simulink model "IEEE34bus_v2019b_Phasor_DPL_ZIPload"  (R2019b)
settings: Solver=VariableStepAuto  StartTime=0.0  StopTime=100  FixedStep=Ts  RelTol=1e-3
InitFcn:
  | a=1; % Loading Factor
  | Ts=0.1;% For Delay Blocks in Voltage Regulator Controls
  | 
  | % Simulation data for the IEEE 34 Node Test Feeder model
  | mi2km = 1.60934;%  miles to km conversion
  | ft2km = 0.0003048; % feet to km conversion
  | ms2F = 1*1e-6/(2*pi*60);% microsiemens to Farads conversion
  | 
  | %% Configuration 300 - series reactance - ohm/mile
  | R_300 = [1.3368 0.2101 0.2130;0.2101 1.3238 0.2066;0.2130 0.2066 1.3294];
  | X_300 = [1.3343 0.5779 0.5015;0.5779 1.3569 0.4591;0.5015 0.4591 1.3471];
  | % charging susceptance - microsiemens/mile
  | B_300 = [5.3350 -1.5313 -0.9943;-1.5313 5.0979 -0.6212;-0.9943 -0.6212 4.8880];
  | 
  | R_300 = R_300/mi2km;
  | L_300 = (X_300/(2*pi*60))/mi2km;
  | C_300 =(B_300*ms2F)/mi2km;
  | 
  | %% Configuration 301 - series reactance - ohm/mile
  | R_301 = [1.9300 0.2327 0.2359;0.2327 1.9157 0.2288;0.2359 0.2288 1.9219];
  | X_301 = [1.4115 0.6442 0.5691;0.6442 1.4281 0.5238;0.5691 0.5238 1.4209];
  | % charging susceptance - microsiemens/mile
  | B_301 = [5.1207 -1.4364 -0.9402;-1.4364 4.9055 -0.5951;-0.9402 -0.5951 4.7154];
  | 
  | R_301 = R_301/mi2km;
  | L_301 = (X_301/(2*pi*60))/mi2km;
  | C_301 =(B_301*ms2F)/mi2km;
  | 
  | 
  | %% Configuration 302 - series reactance - ohm/mile
  | R_302 = [2.7995 0 0;0 0 0;0 0 0];
  | X_302 = [1.4855 0 0;0 0 0;0 0 0];
  | % charging susceptance - microsiemens/mile
  | B_302 = [4.2251 0 0;0 0 0;0 0 0];
  | 
  | R_302 = R_302/mi2km;
  | L_302 = (X_302/(2*pi*60))/mi2km;
  | C_302 =(B_302*ms2F)/mi2km;
  | 
  | %% Configuration 303 - series reactance - ohm/mile
  | R_303 = [0 0 0;0 2.7995 0;0 0 0];
  | X_303 = [0 0 0;0 1.4855 0;0 0 0];
  | % charging susceptance - microsiemens/mile
  | B_303 = [0 0 0;0 4.2251 0;0 0 0];
  | 
  | R_303 = R_303/mi2km;
  | L_303 = (X_303/(2*pi*60))/mi2km;
  | C_303 =(B_303*ms2F)/mi2km;
  | 
  | %% Configuration 303 - series reactance - ohm/mile
  | R_304 = [0 0 0;0 1.9217 0;0 0 0];
  | X_304 = [0 0 0;0 1.4212 0;0 0 0];
  | % charging susceptance - microsiemens/mile
  | B_304 = [0 0 0;0 4.3637 0;0 0 0];
  | 
  | R_304 = R_304/mi2km;
  | L_304 = (X_304/(2*pi*60))/mi2km;
  | C_304 =(B_304*ms2F)/mi2km;
undefined symbols (not defined in the file): find_system, j
libraries: powerlib x471, powerlib_meascontrol x22
(part 9 of 9)

== matlab function IEEE34bus_v2019b_Phasor_DPL_ZIPload/820Y Z/Embedded MATLAB Function ==
  data: Iinj output; Vmeas input; LoadType parameter; Vnom parameter; Pnom parameter; Qnom parameter; Vlim parameter
%Single Phase ZIP Load
%Author: Arun Suresh, University of North Carolina, Charlotte
%Iinj=((Pnom+jQnom)/Vmeas)'
function Iinj = InjectedCurrent(Vmeas,LoadType,Vnom,Pnom,Qnom,Vlim)
% Calculate Pl and Ql.
Kz=0;Ki=0;Kp=0;
Vk=(abs(Vmeas)/Vnom);%(Vmeas/Vnom)
switch LoadType  % 1 for Constant Z, 2 for Constant I and 3 for Constant P, 
    case 1
        Kz=1;
    case 2
        if Vk >= Vlim % convert to Constant Z load due to voltage violation
            Ki=1;
        else
            Kz=1;
        end
    case 3
        if Vk >= Vlim % convert to Constant Z load due to voltage violation
           Kp=1;
        else
            Kz=1;
        end          
 
end
Pl=Pnom *((Kz*Vk*Vk)+(Ki*Vk)+(Kp));
Ql=Qnom *((Kz*Vk*Vk)+(Ki*Vk)+(Kp));
% Net Injected Curent.
% j=sqrt(-1);
Iinj = conj((Pl+j*Ql)/Vmeas);

== matlab function IEEE34bus_v2019b_Phasor_DPL_ZIPload/820 Y PQ/Embedded MATLAB Function ==
  data: Iinj output; Vmeas input; LoadType parameter; Vnom parameter; Pnom parameter; Qnom parameter; Vlim parameter
%Single Phase ZIP Load
%Author: Arun Suresh, University of North Carolina, Charlotte
%Iinj=((Pnom+jQnom)/Vmeas)'
function Iinj = InjectedCurrent(Vmeas,LoadType,Vnom,Pnom,Qnom,Vlim)
% Calculate Pl and Ql.
Kz=0;Ki=0;Kp=0;
Vk=(abs(Vmeas)/Vnom);%(Vmeas/Vnom)
switch LoadType  % 1 for Constant Z, 2 for Constant I and 3 for Constant P, 
    case 1
        Kz=1;
    case 2
        if Vk >= Vlim % convert to Constant Z load due to voltage violation
            Ki=1;
        else
            Kz=1;
        end
    case 3
        if Vk >= Vlim % convert to Constant Z load due to voltage violation
           Kp=1;
        else
            Kz=1;
        end          
 
end
Pl=Pnom *((Kz*Vk*Vk)+(Ki*Vk)+(Kp));
Ql=Qnom *((Kz*Vk*Vk)+(Ki*Vk)+(Kp));
% Net Injected Curent.
% j=sqrt(-1);
Iinj = conj((Pl+j*Ql)/Vmeas);

== matlab function IEEE34bus_v2019b_Phasor_DPL_ZIPload/822 Y PQ/Embedded MATLAB Function ==
  data: Iinj output; Vmeas input; LoadType parameter; Vnom parameter; Pnom parameter; Qnom parameter; Vlim parameter
%Single Phase ZIP Load
%Author: Arun Suresh, University of North Carolina, Charlotte
%Iinj=((Pnom+jQnom)/Vmeas)'
function Iinj = InjectedCurrent(Vmeas,LoadType,Vnom,Pnom,Qnom,Vlim)
% Calculate Pl and Ql.
Kz=0;Ki=0;Kp=0;
Vk=(abs(Vmeas)/Vnom);%(Vmeas/Vnom)
switch LoadType  % 1 for Constant Z, 2 for Constant I and 3 for Constant P, 
    case 1
        Kz=1;
    case 2
        if Vk >= Vlim % convert to Constant Z load due to voltage violation
            Ki=1;
        else
            Kz=1;
        end
    case 3
        if Vk >= Vlim % convert to Constant Z load due to voltage violation
           Kp=1;
        else
            Kz=1;
        end          
 
end
Pl=Pnom *((Kz*Vk*Vk)+(Ki*Vk)+(Kp));
Ql=Qnom *((Kz*Vk*Vk)+(Ki*Vk)+(Kp));
% Net Injected Curent.
% j=sqrt(-1);
Iinj = conj((Pl+j*Ql)/Vmeas);

== matlab function IEEE34bus_v2019b_Phasor_DPL_ZIPload/810 Y I/Embedded MATLAB Function ==
  data: Iinj output; Vmeas input; LoadType parameter; Vnom parameter; Pnom parameter; Qnom parameter; Vlim parameter
%Single Phase ZIP Load
%Author: Arun Suresh, University of North Carolina, Charlotte
%Iinj=((Pnom+jQnom)/Vmeas)'
function Iinj = InjectedCurrent(Vmeas,LoadType,Vnom,Pnom,Qnom,Vlim)
% Calculate Pl and Ql.
Kz=0;Ki=0;Kp=0;
Vk=(abs(Vmeas)/Vnom);%(Vmeas/Vnom)
switch LoadType  % 1 for Constant Z, 2 for Constant I and 3 for Constant P, 
    case 1
        Kz=1;
    case 2
        if Vk >= Vlim % convert to Constant Z load due to voltage violation
            Ki=1;
        else
            Kz=1;
        end
    case 3
        if Vk >= Vlim % convert to Constant Z load due to voltage violation
           Kp=1;
        else
            Kz=1;
        end          
 
end
Pl=Pnom *((Kz*Vk*Vk)+(Ki*Vk)+(Kp));
Ql=Qnom *((Kz*Vk*Vk)+(Ki*Vk)+(Kp));
% Net Injected Curent.
% j=sqrt(-1);
Iinj = conj((Pl+j*Ql)/Vmeas);

== matlab function IEEE34bus_v2019b_Phasor_DPL_ZIPload/808 Y I/Embedded MATLAB Function ==
  data: Iinj output; Vmeas input; LoadType parameter; Vnom parameter; Pnom parameter; Qnom parameter; Vlim parameter
%Single Phase ZIP Load
%Author: Arun Suresh, University of North Carolina, Charlotte
%Iinj=((Pnom+jQnom)/Vmeas)'
function Iinj = InjectedCurrent(Vmeas,LoadType,Vnom,Pnom,Qnom,Vlim)
% Calculate Pl and Ql.
Kz=0;Ki=0;Kp=0;
Vk=(abs(Vmeas)/Vnom);%(Vmeas/Vnom)
switch LoadType  % 1 for Constant Z, 2 for Constant I and 3 for Constant P, 
    case 1
        Kz=1;
    case 2
        if Vk >= Vlim % convert to Constant Z load due to voltage violation
            Ki=1;
        else
            Kz=1;
        end
    case 3
        if Vk >= Vlim % convert to Constant Z load due to voltage violation
           Kp=1;
        else
            Kz=1;
        end          
 
end
Pl=Pnom *((Kz*Vk*Vk)+(Ki*Vk)+(Kp));
Ql=Qnom *((Kz*Vk*Vk)+(Ki*Vk)+(Kp));
% Net Injected Curent.
% j=sqrt(-1);
Iinj = conj((Pl+j*Ql)/Vmeas);
